simulink model "BLDC_FOC_Speed_and_Current_Control"  (R2013a)
settings: Solver=ode45  StartTime=0.0  StopTime=4  RelTol=1e-3
libraries: powerlib x7, powerlib_meascontrol x3, simulink x1
settings Model: Creator=Sony  LastModifiedBy=Sony

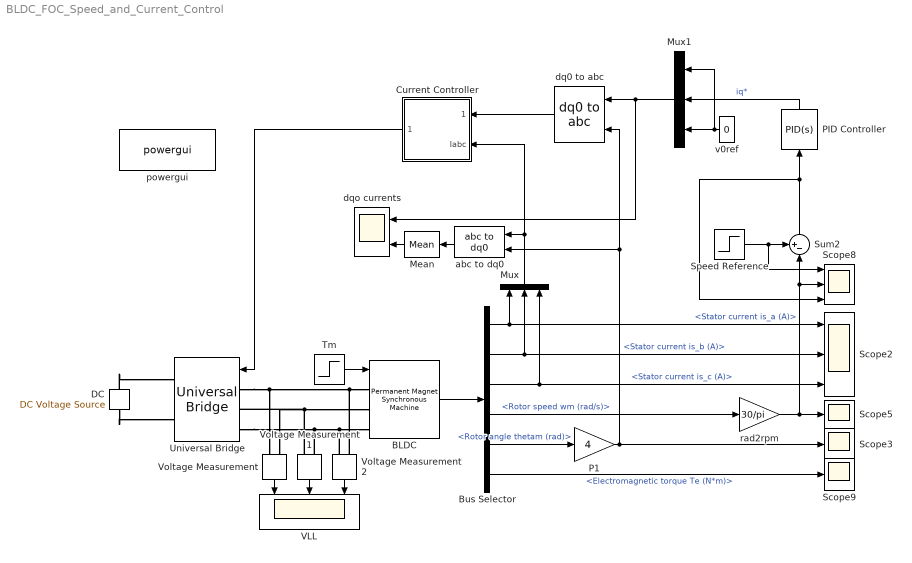
== system BLDC_FOC_Speed_and_Current_Control ==
  BLDC : powerlib/Machines/Permanent Magnet Synchronous Machine  NbPhases=3  FluxDistribution=Trapezoidal  RotorType=Round  MechanicalLoad=Torque Tm  PresetModel=No  ShowDetailedParameters=on  Resistance=0.01  Inductance=1e-4  dqInductances=[8.5e-3,8.5e-3]  La=0.000835  MachineConstant=Flux linkage established by magnets (V.s)  Flux=0.01  VoltageCst=8.3776  TorqueCst=0.08  Flat=120  Mechanical=[1e-3 1e-3 4 0]  PolePairs=4  InitialConditions=[0,0, 0,0]  InitialConditions5ph=[0 0 0 0 0 0]  TsPowergui=0  TsBlock=-1  RefAngle=Aligned with phase A axis (original Park)
  Bus Selector : BusSelector  OutputSignals=Stator current is_a (A),Stator current is_b (A),Stator current is_c (A),Rotor speed wm (rad/s),Rotor angle thetam (rad),Electromagnetic torque Te (N*m)
  Current Controller : Subsystem
  DC : powerlib/Electrical Sources/DC Voltage Source  Amplitude=48  Measurements=None
  Mean : powerlib_meascontrol/Measurements/Mean  Freq=10  Vinit=0  Ts=0
  Mux : Mux  Inputs=3
  Mux1 : Mux  Inputs=3
  P1 : Gain  Gain=4
  PID Controller : simulink/Continuous/PID Controller  Controller=PID  TimeDomain=Continuous-time  SampleTime=1  IntegratorMethod=Forward Euler  FilterMethod=Forward Euler  Form=Parallel  P=1  I=10  D=0  N=100  InitialConditionSource=internal  InitialConditionForIntegrator=0  InitialConditionForFilter=0  ExternalReset=none  LimitOutput=on  UpperSaturationLimit=100  LowerSaturationLimit=-100  LinearizeAsGain=on  AntiWindupMode=clamping  Kb=1  TrackingMode=off  Kt=1  PParamMin=[]  PParamMax=[]  IParamMin=[]  IParamMax=[]  DParamMin=[]  DParamMax=[]  NParamMin=[]  NParamMax=[]  KbParamMin=[]  KbParamMax=[]  KtParamMin=[]  KtParamMax=[]  POutMin=[]  POutMax=[]  IOutMin=[]  IOutMax=[]  DOutMin=[]  DOutMax=[]  NOutMin=[]  NOutMax=[]  KbOutMin=[]  KbOutMax=[]  KtOutMin=[]  KtOutMax=[]  IntegratorOutMin=[]  IntegratorOutMax=[]  FilterOutMin=[]  FilterOutMax=[]  SumOutMin=[]  SumOutMax=[]  SumI1OutMin=[]  SumI1OutMax=[]  SumI2OutMin=[]  SumI2OutMax=[]  SumI3OutMin=[]  SumI3OutMax=[]  SumDOutMin=[]  SumDOutMax=[]  SaturationOutMin=[]  SaturationOutMax=[]  IntegratorContinuousStateAttributes=''  IntegratorStateMustResolveToSignalObject=off  IntegratorRTWStateStorageClass=Auto  FilterContinuousStateAttributes=''  FilterStateMustResolveToSignalObject=off  FilterRTWStateStorageClass=Auto
  Scope2 : Scope  NumInputPorts=3
      settings: YMin=-250~-250~-250  YMax=300~300~300
  Scope3 : Scope
      settings: YMin=0  YMax=7000
  Scope5 : Scope
      settings: YMin=-7000  YMax=7000  SaveName=ScopeData5
  Scope8 : Scope  NumInputPorts=3
      settings: YMin=-3000~-3000~-10  YMax=3000~3000~10  SaveName=ScopeData10
  Scope9 : Scope
      settings: YMin=-10  YMax=10  SaveName=ScopeData11
  Speed Reference : Step  Time=2  Before=-2000  After=2000  SampleTime=0
  Sum2 : Sum  Inputs=+-|
  Tm : Step  Time=2  Before=5  After=5  SampleTime=0
  Universal Bridge : powerlib/Power Electronics/Universal Bridge  Arms=3  SnubberResistance=5000  SnubberCapacitance=1e-6  Device=MOSFET / Diodes  Ron=1e-3  Lon=0  ForwardVoltages="[  0  0  ]"  ForwardVoltage=0  GTOparameters=[ 10e-6 , 20e-6 ]  IGBTparameters=[ 1e-6 , 2e-6 ]  Measurements=None  Measurements_2=None  converterType=Rectifier
  VLL : Scope  NumInputPorts=3
      settings: YMin=-100~-100~-100  YMax=100~100~100  SaveName=ScopeData3
  Voltage Measurement : powerlib/Measurements/Voltage Measurement  PhasorSimulation=off  OutputType=Complex  PSBequivalent=0
  Voltage Measurement1 : powerlib/Measurements/Voltage Measurement  PhasorSimulation=off  OutputType=Complex  PSBequivalent=0
  Voltage Measurement2 : powerlib/Measurements/Voltage Measurement  PhasorSimulation=off  OutputType=Complex  PSBequivalent=0
  abc to dq0 : powerlib_meascontrol/Transformations/abc to dq0  Alignment=Aligned with phase A axis
  dq0 to abc : powerlib_meascontrol/Transformations/dq0 to abc  Alignment=Aligned with phase A axis
  dqo currents : Scope  NumInputPorts=2
      settings: YMin=-10~-10  YMax=110~110  SaveName=ScopeData4
  powergui : powerlib/powergui  Priority=2  SimulationMode=Discrete  SolverType=Backward Euler  SampleTime=1e-5  frequency=60  SPID=off  DisableSnubberDevices=off  DisableRonSwitches=off  DisableVfSwitches=off  SwTol=0  Interpol=off  DisplayEquations=off  frequencyindice=0  Pbase=100e6  ErrMax=1e-4  Iterations=50  UnitsV=kV  UnitsW=MW  FunctionMessages=off  echomessages=off  HookPort=off  EnableUseOfTLC=off  x0status=blocks  RestoreLinks=warning  ResistiveCurrentMeasurement=off  Frange=[0:2:500]  Ylog=off  Xlog=on  ShowGrid=off  save=off  variable=ZData  ZoomFFT=on  StartTime=0.0  cycles=1  DisplayStyle=1  fundamental=60  FreqAxis=off  MaxFrequency=1000  frequencyindicesteady=1  RmsSteady=1  display=off  Ts=0  methode=off
  rad2rpm : Gain  Gain=30/pi
  v0ref : Constant  Value=0
  wires:
  Bus Selector/1 -> Scope2/1, Mux/1  "<Stator current is_a (A)>"
  BLDC/1 -> Bus Selector/1
  Bus Selector/2 -> Scope2/2, Mux/2  "<Stator current is_b (A)>"
  Bus Selector/4 -> rad2rpm/1  "<Rotor speed wm (rad/s)>"
  Bus Selector/3 -> Scope2/3, Mux/3  "<Stator current is_c (A)>"
  Mux/1 -> Current Controller/2(Iabc), abc to dq0/1
  Bus Selector/5 -> P1/1  "<Rotor angle thetam (rad)>"
  Current Controller/1(Pulses) -> Universal Bridge/1
  PID Controller/1 -> Mux1/2  "iq*"
  Mux1/1 -> dqo currents/1, dq0 to abc/1
  v0ref/1 -> Mux1/1, Mux1/3
  P1/1 -> Scope3/1, dq0 to abc/2, abc to dq0/2
  Voltage Measurement2/1 -> VLL/3
  Voltage Measurement1/1 -> VLL/2
  Voltage Measurement/1 -> VLL/1
  Speed Reference/1 -> Scope8/1, Sum2/1
  Sum2/1 -> Scope8/3, PID Controller/1
  dq0 to abc/1 -> Current Controller/1(Iabc_ref)
  rad2rpm/1 -> Scope5/1, Sum2/2, Scope8/2
  Tm/1 -> BLDC/1
  Bus Selector/6 -> Scope9/1  "<Electromagnetic torque Te (N*m)>"
  abc to dq0/1 -> Mean/1
  Mean/1 -> dqo currents/2
  connections:
  Universal Bridge/LConn1 -- Voltage Measurement2/LConn2 -- BLDC/LConn1 -- Voltage Measurement/LConn1
  Universal Bridge/LConn2 -- Voltage Measurement/LConn2 -- Voltage Measurement1/LConn1 -- BLDC/LConn2
  Universal Bridge/LConn3 -- Voltage Measurement1/LConn2 -- Voltage Measurement2/LConn1 -- BLDC/LConn3
  DC/RConn1 -- Universal Bridge/RConn1
  DC/LConn1 -- Universal Bridge/RConn2

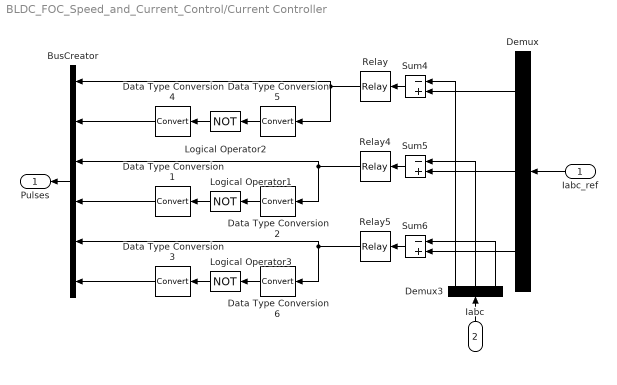
== system BLDC_FOC_Speed_and_Current_Control/Current Controller ==
  Iabc_ref : Inport
  Iabc : Inport  Port=2
  BusCreator : BusCreator  Inputs=6
  Data Type Conversion{1..6} (6 alike) : DataTypeConversion  SaturateOnIntegerOverflow=on  RndMeth=Zero
  Demux : Demux  Outputs=3
  Demux3 : Demux  Outputs=3
  Logical Operator1 : Logic  Operator=NOT
  Logical Operator2 : Logic  Operator=NOT
  Logical Operator3 : Logic  Operator=NOT
  Relay : Relay  OnSwitchValue=1/1000  OffSwitchValue=-1/1000
  Relay4 : Relay  OnSwitchValue=1/1000  OffSwitchValue=-1/1000
  Relay5 : Relay  OnSwitchValue=1/1000  OffSwitchValue=-1/1000
  Sum4 : Sum  Inputs=-+  SaturateOnIntegerOverflow=on  InputSameDT=on  OutDataTypeStr=Inherit: Same as first input
  Sum5 : Sum  Inputs=-+  SaturateOnIntegerOverflow=on  InputSameDT=on  OutDataTypeStr=Inherit: Same as first input
  Sum6 : Sum  Inputs=-+  SaturateOnIntegerOverflow=on  InputSameDT=on  OutDataTypeStr=Inherit: Same as first input
  Pulses : Outport
  wires:
  Iabc/1 -> Demux3/1
  Demux/2 -> Sum5/2
  Demux/1 -> Sum4/2
  Sum4/1 -> Relay/1
  Demux3/2 -> Sum5/1
  Demux3/1 -> Sum4/1
  Sum5/1 -> Relay4/1
  Demux3/3 -> Sum6/1
  Demux/3 -> Sum6/2
  Sum6/1 -> Relay5/1
  Iabc_ref/1 -> Demux/1
  Logical Operator2/1 -> Data Type Conversion4/1
  Data Type Conversion5/1 -> Logical Operator2/1
  Relay/1 -> BusCreator/1, Data Type Conversion5/1
  Data Type Conversion4/1 -> BusCreator/2
  Logical Operator1/1 -> Data Type Conversion1/1
  Data Type Conversion2/1 -> Logical Operator1/1
  Data Type Conversion1/1 -> BusCreator/4
  Logical Operator3/1 -> Data Type Conversion3/1
  Data Type Conversion6/1 -> Logical Operator3/1
  Data Type Conversion3/1 -> BusCreator/6
  Relay4/1 -> BusCreator/3, Data Type Conversion2/1
  Relay5/1 -> BusCreator/5, Data Type Conversion6/1
  BusCreator/1 -> Pulses/1
